simulink model "DAB"  (R2024b)
settings: Solver=VariableStepAuto  StartTime=0.0  StopTime=0.01  RelTol=1e-3
libraries: spsSeriesRLCBranchLib x9, spsMosfetLib x8, spsDCVoltageSourceLib x2, spsVoltageMeasurementLib x2, spsLinearTransformerLib x1, sps_lib x1
settings Model: Creator=wei13  LastModifiedBy=wei13

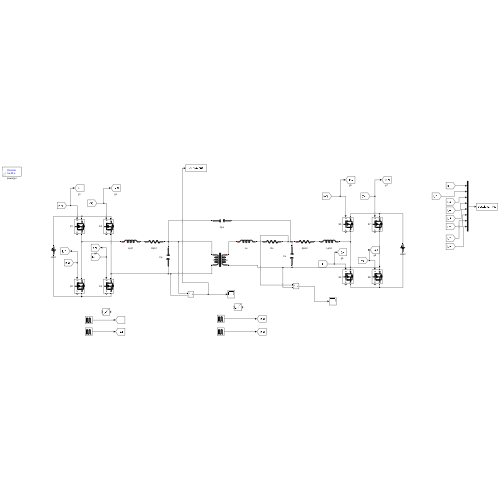
[thumbnail: Simulink's stored preview of the top-level diagram]
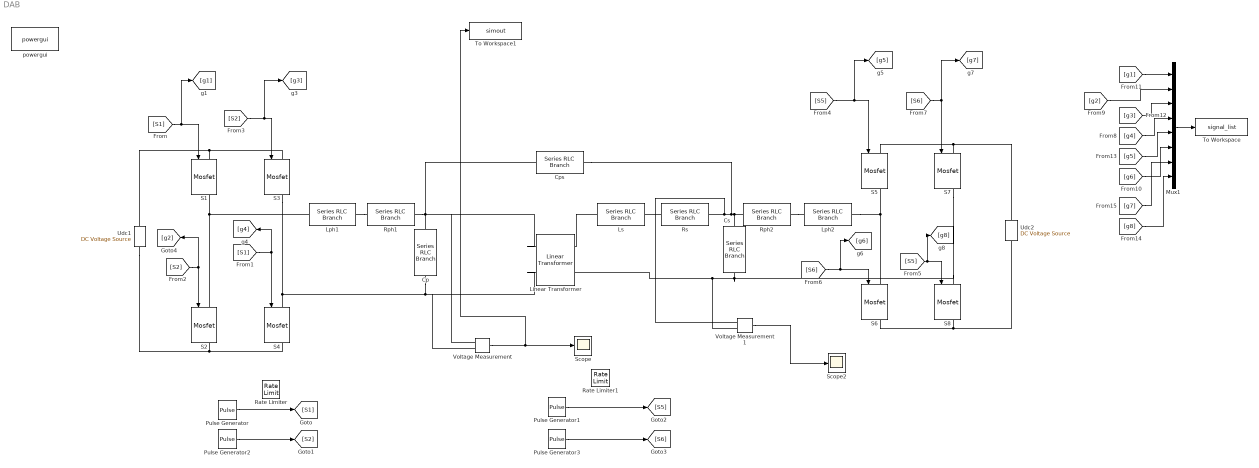
== system DAB ==
  Cp : spsSeriesRLCBranchLib/Series RLC Branch  LConnTagsString=__new0  RConnTagsString=__new0  BranchType=C  Resistance=1  Inductance=0  SetiL0=off  InitialCurrent=0  Capacitance=39.1e-12  Setx0=off  InitialVoltage=0  Measurements=None
  Cps : spsSeriesRLCBranchLib/Series RLC Branch  LConnTagsString=__new0  RConnTagsString=__new0  BranchType=C  Resistance=1  Inductance=0  SetiL0=off  InitialCurrent=0  Capacitance=129e-12  Setx0=off  InitialVoltage=0  Measurements=None
  Cs : spsSeriesRLCBranchLib/Series RLC Branch  LConnTagsString=__new0  RConnTagsString=__new0  BranchType=C  Resistance=1  Inductance=0  SetiL0=off  InitialCurrent=0  Capacitance=39.1e-12  Setx0=off  InitialVoltage=0  Measurements=None
  Linear Transformer : spsLinearTransformerLib/Linear Transformer  UNITS=SI  NominalPower=[ 250e6 10000]  winding1=[600 0 0]  winding2=[600 0 0]  ThreeWindings=off  winding3=[3.15e+05 0.7938 0.084225]  RmLm=[12e3 63e-3]  Measurements=None  DataType=on
  Lph1 : spsSeriesRLCBranchLib/Series RLC Branch  LConnTagsString=__new0  RConnTagsString=__new0  BranchType=L  Resistance=1  Inductance=60.51e-6  SetiL0=off  InitialCurrent=0  Capacitance=Inf  Setx0=off  InitialVoltage=0  Measurements=None
  Lph2 : spsSeriesRLCBranchLib/Series RLC Branch  LConnTagsString=__new0  RConnTagsString=__new0  BranchType=L  Resistance=1  Inductance=60.51e-6  SetiL0=off  InitialCurrent=0  Capacitance=Inf  Setx0=off  InitialVoltage=0  Measurements=None
  Ls : spsSeriesRLCBranchLib/Series RLC Branch  LConnTagsString=__new0  RConnTagsString=__new0  BranchType=L  Resistance=1  Inductance=5.1e-6  SetiL0=off  InitialCurrent=0  Capacitance=Inf  Setx0=off  InitialVoltage=0  Measurements=None
  Mux1 : Mux  Inputs=8
  Pulse Generator : DiscretePulseGenerator  PulseType=Time based  Period=100e-6  PulseWidth=50
  Pulse Generator1 : DiscretePulseGenerator  PulseType=Time based  Period=100e-6  PulseWidth=50  PhaseDelay=25e-6
  Pulse Generator2 : DiscretePulseGenerator  PulseType=Time based  Period=100e-6  PulseWidth=50  PhaseDelay=50e-6
  Pulse Generator3 : DiscretePulseGenerator  PulseType=Time based  Period=100e-6  PulseWidth=50  PhaseDelay=75e-6
  Rate Limiter : RateLimiter  RisingSlewLimit=4.6e10  FallingSlewLimit=-4.6e10
  Rate Limiter1 : RateLimiter  RisingSlewLimit=4.6e10  FallingSlewLimit=-4.6e10
  Rph1 : spsSeriesRLCBranchLib/Series RLC Branch  LConnTagsString=__new0  RConnTagsString=__new0  BranchType=R  Resistance=0.016  Inductance=0  SetiL0=off  InitialCurrent=0  Capacitance=Inf  Setx0=off  InitialVoltage=0  Measurements=None
  Rph2 : spsSeriesRLCBranchLib/Series RLC Branch  LConnTagsString=__new0  RConnTagsString=__new0  BranchType=R  Resistance=0.016  Inductance=0  SetiL0=off  InitialCurrent=0  Capacitance=Inf  Setx0=off  InitialVoltage=0  Measurements=None
  Rs : spsSeriesRLCBranchLib/Series RLC Branch  LConnTagsString=__new0  RConnTagsString=__new0  BranchType=R  Resistance=0.04  Inductance=0  SetiL0=off  InitialCurrent=0  Capacitance=Inf  Setx0=off  InitialVoltage=0  Measurements=None
  S{1..4} (4 alike) : spsMosfetLib/Mosfet  Ron=0.1  Lon=0  Rd=0.01  Vfd=0  IC=0  Rs=1e5  Cs=Inf  Measurements=on
  S{5..8} (4 alike) : spsMosfetLib/Mosfet  Ron=0.1  Lon=0  Rd=0.01  Vfd=0  IC=0  Rs=1e5  Cs=inf  Measurements=on
  Scope : Scope
  Scope2 : Scope
  To Workspace : ToWorkspace  VariableName=signal_list  SampleTime=-1
      settings: Save2DSignal=2-D array (concatenate along first dimension)
  To Workspace1 : ToWorkspace  VariableName=simout  SaveFormat=Timeseries  SampleTime=-1
  Udc1 : spsDCVoltageSourceLib/DC Voltage Source  Amplitude=600  Measurements=None
  Udc2 : spsDCVoltageSourceLib/DC Voltage Source  Amplitude=600  Measurements=None
  Voltage Measurement : spsVoltageMeasurementLib/Voltage Measurement  PhasorSimulation=off  OutputType=Complex  PSBequivalent=0
  Voltage Measurement1 : spsVoltageMeasurementLib/Voltage Measurement  PhasorSimulation=off  OutputType=Complex  PSBequivalent=0
  powergui : sps_lib/powergui  Priority=1  SimulationMode=Discrete  SampleTime=5e-8  frequency=60  Iterations=50  frequencyindice=0  Pbase=100e6  ErrMax=1e-4  UnitsV=kV  UnitsW=MW  buscounter=0  FunctionMessages=off  echomessages=off  EnableUseOfTLC=off  CurrentSourceSwitches=off  DisableSnubberDevices=off  DisableRonSwitches=off  DisableVfSwitches=off  DisplayEquations=off  AutomaticDiscreteSolvers=off  SolverType=Tustin/Backward Euler (TBE)  Interpol=off  ExternalGateDelay=off  methode=off  Ts=100  x0status=blocks  SPID=on  SwTol=0  HookPort=off  NonlinearTolerance=1e-4  nMaxIteration=100  ContinueOnMaxIteration=off  RestoreLinks=warning  ResistiveCurrentMeasurement=off  Frange=[0:2:500]  Ylog=off  Xlog=on  ShowGrid=off  save=off  variable=ZData  structure=0  ZoomFFT=off  StartTime=0.0  cycles=1  DisplayStyle=1  fundamental=60  FreqAxis=off  MaxFrequency=1000  frequencyindicesteady=1  RmsSteady=1  display=off
  wires:
  Voltage Measurement/1 -> To Workspace1/1, Scope/1
  [S1] -> [g1], S1/1
  [S1] -> [g4], S4/1
  [S2] -> [g2], S2/1
  [S2] -> [g3], S3/1
  [S5] -> [g5], S5/1
  [S5] -> [g8], S8/1
  [S6] -> [g6], S6/1
  [S6] -> [g7], S7/1
  Voltage Measurement1/1 -> Scope2/1
  Pulse Generator/1 -> [S1]
  Pulse Generator1/1 -> [S5]
  [g1] -> Mux1/1
  [g2] -> Mux1/2
  [g3] -> Mux1/3
  Mux1/1 -> To Workspace/1
  [g6] -> Mux1/6
  [g4] -> Mux1/4
  [g5] -> Mux1/5
  [g7] -> Mux1/7
  [g8] -> Mux1/8
  Pulse Generator2/1 -> [S2]
  Pulse Generator3/1 -> [S6]
  connections:
  Rph1/RConn1 -- Voltage Measurement/LConn1 -- Linear Transformer/LConn1 -- Cps/LConn1 -- Cp/LConn1
  Lph1/RConn1 -- Rph1/LConn1
  Ls/LConn1 -- Linear Transformer/RConn1
  Rs/LConn1 -- Ls/RConn1
  Cs/LConn1 -- Cps/RConn1 -- Voltage Measurement1/LConn1 -- Rs/RConn1 -- Rph2/LConn1
  Rph2/RConn1 -- Lph2/LConn1
  Lph1/LConn1 -- S2/LConn1 -- S1/RConn1
  S2/RConn1 -- Udc1/LConn1 -- S4/RConn1
  S3/LConn1 -- Udc1/RConn1 -- S1/LConn1
  S5/LConn1 -- Udc2/RConn1 -- S7/LConn1
  S6/RConn1 -- Udc2/LConn1 -- S8/RConn1
  S6/LConn1 -- S5/RConn1 -- Lph2/RConn1
  Cs/RConn1 -- S7/RConn1 -- S8/LConn1 -- Voltage Measurement1/LConn2 -- Linear Transformer/RConn2
  S3/RConn1 -- Voltage Measurement/LConn2 -- Linear Transformer/LConn2 -- Cp/RConn1 -- S4/LConn1
